simulink model "OOCconSistemaSeguimientoSinIntegrador"  (R2020a)
settings: Solver=VariableStepAuto  StartTime=0.0  StopTime=10  RelTol=1e-3
settings Model: Creator=Sergio  LastModifiedBy=Sergio

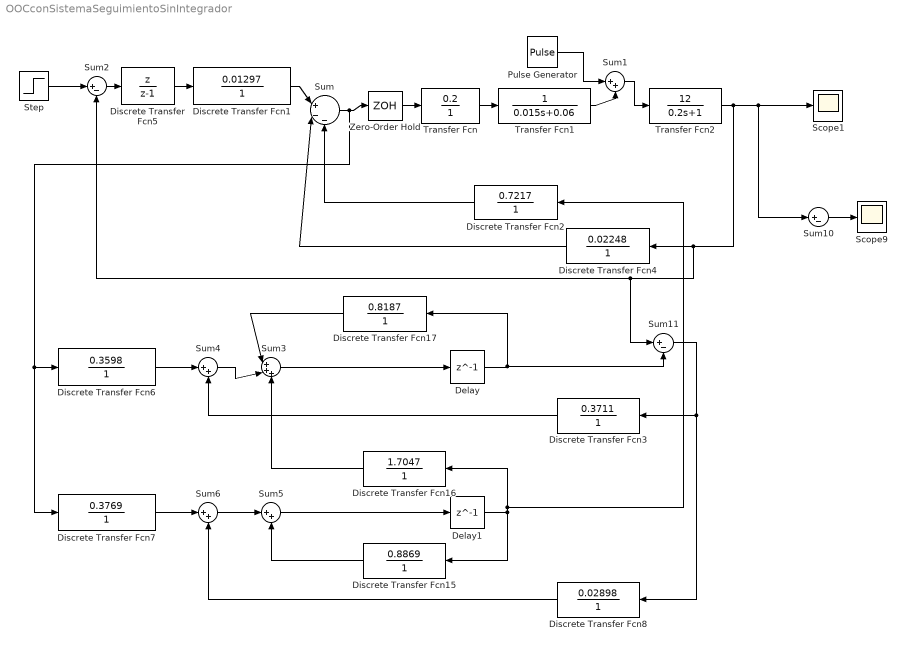
== system OOCconSistemaSeguimientoSinIntegrador ==
  Delay : Delay  DelayLength=1
  Delay1 : Delay  DelayLength=1
  Discrete Transfer Fcn1 : DiscreteTransferFcn  Numerator=[0.01297]  Denominator=[1]
  Discrete Transfer Fcn15 : DiscreteTransferFcn  Numerator=[0.8869]  Denominator=[1]
  Discrete Transfer Fcn16 : DiscreteTransferFcn  Numerator=[1.7047]  Denominator=[1]
  Discrete Transfer Fcn17 : DiscreteTransferFcn  Numerator=[0.8187]  Denominator=[1]
  Discrete Transfer Fcn2 : DiscreteTransferFcn  Numerator=[0.7217]  Denominator=[1]
  Discrete Transfer Fcn3 : DiscreteTransferFcn  Numerator=[0.3711]  Denominator=[1]
  Discrete Transfer Fcn4 : DiscreteTransferFcn  Numerator=[0.02248]  Denominator=[1]
  Discrete Transfer Fcn5 : DiscreteTransferFcn  Numerator=[1 0]  Denominator=[1 -1]
  Discrete Transfer Fcn6 : DiscreteTransferFcn  Numerator=[0.3598]  Denominator=[1]
  Discrete Transfer Fcn7 : DiscreteTransferFcn  Numerator=[0.3769]  Denominator=[1]
  Discrete Transfer Fcn8 : DiscreteTransferFcn  Numerator=[0.02898]  Denominator=[1]
  Pulse Generator : DiscretePulseGenerator  PulseType=Time based  Amplitude=0.1  Period=10
  Scope1 : Scope
  Scope9 : Scope
  Step : Step  SampleTime=0
  Sum : Sum  Inputs=|+--
  Sum{1,4..6} (4 alike) : Sum  Inputs=|++
  Sum10 : Sum  Inputs=|+-
  Sum11 : Sum  Inputs=|+-
  Sum2 : Sum  Inputs=|+-
  Sum3 : Sum  Inputs=|+++
  Transfer Fcn : TransferFcn  Numerator=[0.2]  Denominator=[1]
  Transfer Fcn1 : TransferFcn  Denominator=[0.015 0.06]
  Transfer Fcn2 : TransferFcn  Numerator=[12]  Denominator=[0.2 1]
  Zero-Order Hold : ZeroOrderHold  SampleTime=0.04
  wires:
  Zero-Order Hold/1 -> Transfer Fcn/1
  Sum/1 -> Discrete Transfer Fcn7/1, Discrete Transfer Fcn6/1, Zero-Order Hold/1
  Transfer Fcn2/1 -> Discrete Transfer Fcn4/1, Sum11/1, Sum2/2, Sum10/1, Scope1/1
  Transfer Fcn1/1 -> Sum1/2
  Sum1/1 -> Transfer Fcn2/1
  Transfer Fcn/1 -> Transfer Fcn1/1
  Discrete Transfer Fcn2/1 -> Sum/3
  Pulse Generator/1 -> Sum1/1
  Step/1 -> Sum2/1
  Discrete Transfer Fcn1/1 -> Sum/1
  Discrete Transfer Fcn5/1 -> Discrete Transfer Fcn1/1
  Sum2/1 -> Discrete Transfer Fcn5/1
  Discrete Transfer Fcn4/1 -> Sum/2
  Discrete Transfer Fcn6/1 -> Sum4/1
  Discrete Transfer Fcn7/1 -> Sum6/1
  Sum4/1 -> Sum3/2
  Sum3/1 -> Delay/1
  Delay/1 -> Sum11/2, Discrete Transfer Fcn17/1
  Discrete Transfer Fcn17/1 -> Sum3/1
  Sum5/1 -> Delay1/1
  Delay1/1 -> Discrete Transfer Fcn2/1, Discrete Transfer Fcn16/1, Discrete Transfer Fcn15/1
  Discrete Transfer Fcn16/1 -> Sum3/3
  Sum10/1 -> Scope9/1
  Discrete Transfer Fcn15/1 -> Sum5/2
  Sum6/1 -> Sum5/1
  Sum11/1 -> Discrete Transfer Fcn8/1, Discrete Transfer Fcn3/1
  Discrete Transfer Fcn3/1 -> Sum4/2
  Discrete Transfer Fcn8/1 -> Sum6/2
